simulink model "kinect_kalman_test"  (R2015b)
settings: Solver=VariableStepAuto  StartTime=0.0  StopTime=10  RelTol=1e-3
values from neighbouring files (symbols this model uses):
  filterOrder = 10    [init_kinect_kalman.m]
  freq = 0.4    [init_kinect_kalman.m]
  std_R = [0.1]    [init_kinect_kalman.m]
undefined symbols (not defined in the file or in its folder): KFparam
settings Model: Creator=mgreiff  LastModifiedBy=mgreiff

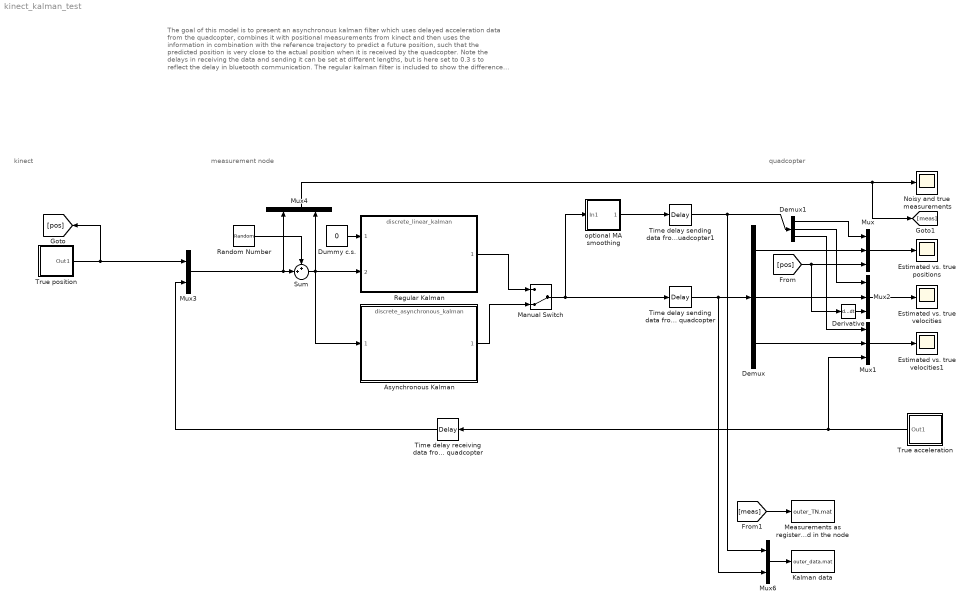
== system kinect_kalman_test ==
  note: The goal of this model is to present an asynchronous kalman filter which uses delayed
      | acceleration data from the quadcopter, combines it with positional measurements from
      | kinect and then uses the information in combination with the reference trajectory to predict
      | a future position, such that the predicted position is very close to the actual position when it
      | is received by the quadcopter. Note the delays in receiving the data and sending it can be
      | set at different lengths, but is here set to 0.3 s to reflect the delay in bluetooth communication.
      | The regular kalman filter is included to show the difference in filtering.
  note: kinect
  note: quadcopter
  note: measurement node
  Asynchronous Kalman : ModelReference  ModelNameDialog=discrete_asynchronous_kalman.slx  SimulationMode=Normal  ModelReferenceVersion=1.92  CopyOfModelName=discrete_asynchronous_kalman.slx
  Demux : Demux  Outputs=[1,1,1]
  Demux1 : Demux  Outputs=[1,1,1]
  Derivative : Derivative
  Dummy c.s. : Constant  Value=0
  Estimated vs. true positions : Scope
  Estimated vs. true velocities : Scope
  Estimated vs. true velocities1 : Scope
  Kalman data : ToFile  Filename=outer_data.mat  MatrixName=AKF  SaveFormat=Timeseries
  Manual Switch : ManualSwitch  CurrentSetting=0
  Measurements as registered in the node : ToFile  Filename=outer_TN.mat  MatrixName=TN  SaveFormat=Timeseries
  Mux : Mux  Inputs=3
  Mux1 : Mux  Inputs=3
  Mux2 : Mux  Inputs=3
  Mux3 : Mux  Inputs=2
  Mux4 : Mux  Inputs=2
  Mux6 : Mux  Inputs=2
  Noisy and true measurements : Scope
  Random Number : RandomNumber  Mean=std_R.*0  Variance=std_R.^2  SampleTime=KFparam.h
  Regular Kalman : ModelReference  ModelNameDialog=discrete_linear_kalman.slx  SimulationMode=Normal  ModelReferenceVersion=1.90  CopyOfModelName=discrete_linear_kalman.slx
  Sum : Sum  Inputs=++|
  Time delay receiving data from quadcopter : TransportDelay  DelayTime=KFparam.recDelay
  Time delay sending data from quadcopter : TransportDelay  DelayTime=KFparam.sendDelay
  Time delay sending data from quadcopter1 : TransportDelay  DelayTime=KFparam.sendDelay
  True acceleration : Subsystem
  True position : Subsystem
  optional MA smoothing : Subsystem
  wires:
  Dummy c.s./1 -> Regular Kalman/1
  Mux/1 -> Estimated vs. true positions/1
  Sum/1 -> Asynchronous Kalman/1, Regular Kalman/2, Mux4/2
  Random Number/1 -> Sum/1
  Mux1/1 -> Estimated vs. true velocities1/1
  Demux/3 -> Mux1/2
  Demux/1 -> Mux/2
  Demux/2 -> Mux2/2
  Demux1/1 -> Mux/1
  Mux2/1 -> Estimated vs. true velocities/1
  Demux1/2 -> Mux2/1
  Demux1/3 -> Mux1/1
  Mux3/1 -> Sum/2, Mux4/1
  Mux4/1 -> [meas], Noisy and true measurements/1
  True acceleration/1(Out1) -> Time delay receiving data from quadcopter/1, Mux1/3
  [pos] -> Derivative/1, Mux/3
  Derivative/1 -> Mux2/3
  optional MA smoothing/1(Out1) -> Time delay sending data from quadcopter1/1
  Asynchronous Kalman/1 -> Manual Switch/2
  Manual Switch/1 -> optional MA smoothing/1(In1), Time delay sending data from quadcopter/1
  Time delay sending data from quadcopter1/1 -> Mux6/1, Demux1/1
  True position/1(Out1) -> Mux3/1, [pos]
  Regular Kalman/1 -> Manual Switch/1
  Mux6/1 -> Kalman data/1
  Time delay sending data from quadcopter/1 -> Mux6/2, Demux/1
  [meas] -> Measurements as registered in the node/1
  Time delay receiving data from quadcopter/1 -> Mux3/2

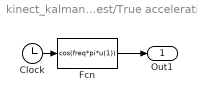
== system kinect_kalman_test/True acceleration ==
  Clock : Clock
  Fcn : Fcn  Expr=cos(freq*pi*u(1))
  Out1 : Outport
  wires:
  Fcn/1 -> Out1/1
  Clock/1 -> Fcn/1

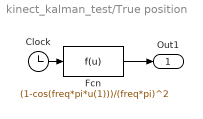
== system kinect_kalman_test/True position ==
  Clock : Clock
  Fcn : Fcn  Expr=(1-cos(freq*pi*u(1)))/(freq*pi)^2
  Out1 : Outport
  wires:
  Fcn/1 -> Out1/1
  Clock/1 -> Fcn/1

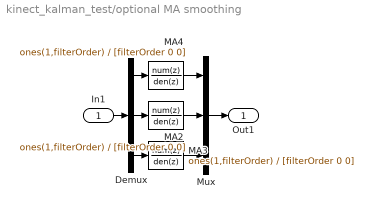
== system kinect_kalman_test/optional MA smoothing ==
  In1 : Inport
  Demux : Demux  Outputs=3
  MA2 : DiscreteFilter  Numerator=ones(1,filterOrder)  Denominator=[filterOrder 0 0]
  MA3 : DiscreteFilter  Numerator=ones(1,filterOrder)  Denominator=[filterOrder 0 0]
  MA4 : DiscreteFilter  Numerator=ones(1,filterOrder)  Denominator=[filterOrder 0 0]
  Mux : Mux  Inputs=3
  Out1 : Outport
  wires:
  Demux/3 -> MA3/1
  Demux/2 -> MA2/1
  Demux/1 -> MA4/1
  MA4/1 -> Mux/1
  MA2/1 -> Mux/2
  MA3/1 -> Mux/3
  Mux/1 -> Out1/1
  In1/1 -> Demux/1
